simulink model "car_trailer_parking_model"  (R2024b)
settings: Solver=ode15s  StartTime=0.0  StopTime=5  FixedStep=1e-6  MaxStep=0.1  RelTol=1e-3  AbsTol=1e-6
undefined symbols (not defined in the file): Ion, Lithium, ref_traj_parking, ref_traj_reverse, ref_traj_straight
libraries: autolibshared x2, slpidlib x2, spsBatteryLib x1, spsDCMachineLib x1, spsGroundLib x1, spsFullBridgeMMCLib x1, spsPWMGenerator2LevelLib x1, vehdynlibeom x1, spsVariableCapacitorLib x1, spsVariableResistorLib x1, spspowerguiLib x1
(part 2 of 2)

== matlab function car_trailer_parking_model/MATLAB Function1 ==
  data: manselect input; port_index output
function port_index = map_manselect(manselect)
        switch manselect
            case {1, 4}
                port_index = 1; % TrajParking
            case {2, 5}
                port_index = 2; % TrajStraight
            case {3, 6}
                port_index = 3; % TrajReverse
            otherwise
                port_index = 2; % Default to TrajStraight
        end
    end

== matlab function car_trailer_parking_model/MATLAB Function ==
  data: x_c input double size=1; delta output double size=1; y_c input double size=1; theta_c input double size=1; ref_traj input double size=[50, 3]; L_d input double size=1; L_c input double size=1; manselect input
function delta = PurePursuit(x_c, y_c, theta_c, ref_traj, L_d, L_c, manselect)
    % Initialize default goal
    goal_x = ref_traj(end, 1);
    goal_y = ref_traj(end, 2);

    % Force delta = 0 for straight and reverse maneuvers
    if ismember(manselect, [2, 3, 5, 6])
        delta = 0;
        return;
    end

    % Find closest point on reference trajectory
    distances = sqrt((ref_traj(:,1) - x_c).^2 + (ref_traj(:,2) - y_c).^2);
    [~, idx] = min(distances);

    % Lookahead point
    for i = idx:length(ref_traj)
        if distances(i) >= L_d
            goal_x = ref_traj(i, 1);
            goal_y = ref_traj(i, 2);
            break;
        end
    end

    % Calculate steering angle
    alpha = atan2(goal_y - y_c, goal_x - x_c) - theta_c;
    alpha = mod(alpha + pi, 2*pi) - pi; % Normalize to [-pi, pi]
    delta = atan2(2 * L_c * sin(alpha), L_d);

    % Clamp delta
    delta = max(min(delta, 0.5236), -0.5236);
end

== matlab function car_trailer_parking_model/MATLAB Function2 ==
  data: CarVelocity input double size=1; XVelocity output double size=1; SteeringAngle input double size=1; CarOrientation input double size=1; TrailerOrientation input double size=1; YVelocity output double size=1; CarOrientationChange output double size=1; TrailerOrientationChange output double size=1; TrailerEnable input; manselect input
function [XVelocity, YVelocity, CarOrientationChange, TrailerOrientationChange] = CarKinematics(CarVelocity, SteeringAngle, CarOrientation, TrailerOrientation, TrailerEnable, manselect)
    persistent CarLength TrailerLength HitchLength Factor;
    if isempty(CarLength)
        CarLength = 4; % meters
        TrailerLength = 6; % meters
        HitchLength = 1; % meters
        Factor = CarLength / (CarLength + HitchLength);
    end

    % Clamp SteeringAngle
    SteeringAngle = max(min(SteeringAngle, 0.5236), -0.5236);

    % Velocity at car center (CarVelocity is speed at front)
    XVelocity = CarVelocity * cos(CarOrientation);
    YVelocity = CarVelocity * sin(CarOrientation);
    CarOrientationChange = (CarVelocity / CarLength) * tan(SteeringAngle);

    % Trailer dynamics
    if TrailerEnable == 1
        RelativeAngle = CarOrientation - TrailerOrientation;
        TrailerOrientationChange = (CarVelocity / TrailerLength) * sin(RelativeAngle) * Factor;
    else
        TrailerOrientationChange = 0; % No trailer dynamics
    end

    % Commented overrides for potential reversion
    %{
    % Overrides for straight maneuvers (manselect = 2, 5)
    if manselect == 2 || manselect == 5
        YVelocity = 0; % No lateral motion
        CarOrientationChange = 0; % No orientation change
        TrailerOrientationChange = 0; % No trailer rotation
        return;
    end

    % Overrides for reverse maneuvers (manselect = 3, 6)
    if manselect == 3 || manselect == 6
        YVelocity = 0; % No lateral motion
        CarOrientationChange = 0; % No orientation change
        TrailerOrientationChange = 0; % No trailer rotation
        return;
    end
    %}
end

== matlab function car_trailer_parking_model/MATLAB Function3 ==
  data: TrailerEnable input; Fz output; Fh output
function [Fz, Fh] = TrailerEnableSwitch(TrailerEnable)
    if TrailerEnable == 1
        Fz = 22600; % Fz with trailer
        Fh = [981, 0, 9810]; % Hitch force with trailer
    else
        Fz = 20600; % Fz without trailer
        Fh = [0, 0, 0]; % No hitch force
    end
end
